simulink model "chap9_5sim"  (Simulink 5.0)
settings: Solver=ode45  StartTime=0.0  StopTime=20  FixedStep=0.001  RelTol=1e-3
settings Model: LastModifiedBy=ljk  ExtModeTrigMode=oneshot  ExtModeArmWhenConnect=off  LimitDataPoints=off  BooleanDataType=off

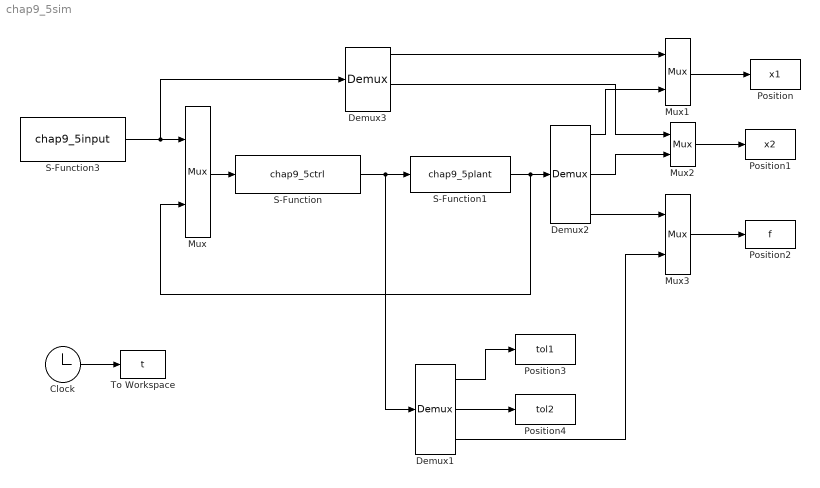
== system chap9_5sim ==
  Clock : Clock
      settings: Decimation=10
  Demux1 : Demux  Outputs=3
  Demux2 : Demux  Outputs=5
  Demux3 : Demux  Outputs=6
  Mux{,1..3} (4 alike) : Mux  Inputs=2
  Position : ToWorkspace  VariableName=x1  SampleTime=-1  SaveFormat=Array
  Position1 : ToWorkspace  VariableName=x2  SampleTime=-1  SaveFormat=Array
  Position2 : ToWorkspace  VariableName=f  SampleTime=-1  SaveFormat=Array
  Position3 : ToWorkspace  VariableName=tol1  SampleTime=-1  SaveFormat=Array
  Position4 : ToWorkspace  VariableName=tol2  SampleTime=-1  SaveFormat=Array
  S-Function : S-Function  FunctionName=chap9_5ctrl
  S-Function1 : S-Function  FunctionName=chap9_5plant
  S-Function3 : S-Function  FunctionName=chap9_5input
  To Workspace : ToWorkspace  VariableName=t  SampleTime=-1  SaveFormat=Array
  wires:
  Mux/1 -> S-Function/1
  Demux2/1 -> Mux1/2
  S-Function1/1 -> Demux2/1, Mux/2
  Demux1/1 -> Position3/1
  Demux1/2 -> Position4/1
  Demux3/1 -> Mux1/1
  Mux1/1 -> Position/1
  Mux2/1 -> Position1/1
  S-Function/1 -> S-Function1/1, Demux1/1
  Mux3/1 -> Position2/1
  Demux1/3 -> Mux3/2
  Demux2/5 -> Mux3/1
  Demux3/4 -> Mux2/1
  Demux2/3 -> Mux2/2
  Clock/1 -> To Workspace/1
  S-Function3/1 -> Mux/1, Demux3/1
